simulink model "Schwinger_V1"  (R2016a)
settings: Solver=ode1  StartTime=0.0  StopTime=1000  FixedStep=0.01  RelTol=1e-3
undefined symbols (not defined in the file): delta, omega
settings Model: Creator=Michaél  LastModifiedBy=Michaél

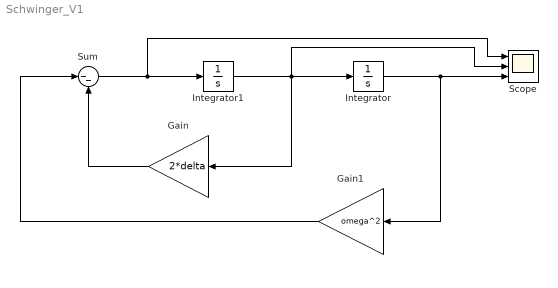
== system Schwinger_V1 ==
  Gain : Gain  Gain=2*delta
  Gain1 : Gain  Gain=omega^2
  Integrator : Integrator  InitialCondition=5
  Integrator1 : Integrator
  Scope : Scope  NumInputPorts=3
  Sum : Sum  Inputs=|--
  wires:
  Gain/1 -> Sum/2
  Gain1/1 -> Sum/1
  Integrator/1 -> Scope/3, Gain1/1
  Integrator1/1 -> Gain/1, Scope/2, Integrator/1
  Sum/1 -> Scope/1, Integrator1/1
